simulink model "gm_FFT_DUT"  (R2021a)
settings: Solver=FixedStepDiscrete  StartTime=0.0  StopTime=54  RelTol=1e-3
libraries: simulink x1, dsphdlxfrm x1, dspsrcs4 x1
settings Model: Creator=Tood  LastModifiedBy=Tood
settings SolverCC: AlgebraicLoopSolver=TrustRegion
settings DataIOCC: LimitDataPoints=on  SaveOutput=off  SaveTime=off
settings OptimizationCC: BlockReduction=off  ConditionallyExecuteInputs=off  DefaultParameterBehavior=Inlined  LifeSpan=inf
settings DebuggingCC: AlgebraicLoopMsg=error  InheritedTsInSrcMsg=none  SingleTaskRateTransMsg=error  AllowSymbolicDim=off  StrictBusMsg=ErrorOnBusTreatedAsVector  SFUnexpectedBacktrackingDiag=warning  SFNoUnconditionalDefaultTransitionDiag=warning  SFExecutionAtInitializationDiag=none  SFMachineParentedDataDiag=warning  ArithmeticOperatorsInVariantConditions=warning
settings HardwareCC: ProdBitPerPointer=32  ProdBitPerSizeT=32  ProdBitPerPtrDiffT=32  ProdLargestAtomicFloat=None  ProdIntDivRoundTo=Undefined  ProdEndianess=Unspecified  ProdWordSize=32  ProdHWDeviceType=ASIC/FPGA->ASIC/FPGA  TargetBitPerPointer=64  TargetBitPerSizeT=64  TargetBitPerPtrDiffT=64  TargetLongLongMode=on  TargetIntDivRoundTo=Zero  TargetEndianess=LittleEndian  TargetWordSize=64  TargetHWDeviceType=Custom Processor->MATLAB Host Computer  ProdEqTarget=off
settings SFSimCC: SimUseLocalCustomCode=off  CustomCodeUndefinedFunction=UseInterfaceOnly
settings RTWCC: RTWUseLocalCustomCode=off
settings CodeAppCC: StateflowObjectComments=on
settings GRTTargetCC: TargetLangStandard=C89/C90 (ANSI)
settings ConfigComp: CovScope=ReferencedModels  CovMetricSettings=dw  CovSaveCumulativeToWorkspaceVar=on  CovSaveSingleToWorkspaceVar=on  CovExternalEMLEnable=off  CovSFcnEnable=off

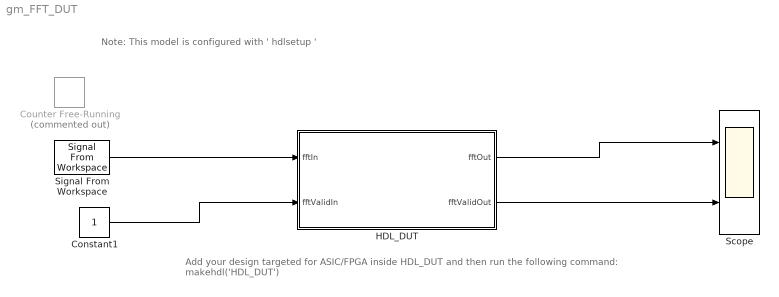
== system gm_FFT_DUT ==
  note: Add your design targeted for ASIC/FPGA inside HDL_DUT and then run the following command:
      | makehdl('HDL_DUT')
  note: Note: This model is configured with ' hdlsetup '
  Constant1 : Constant  OutDataTypeStr=boolean  SampleTime=-1
  Counter Free-Running : simulink/Sources/Counter Free-Running  Commented=on  NumBits=16  tsamp=-1
  HDL_DUT : Subsystem
  Scope : Scope  NumInputPorts=2
  Signal From Workspace : dspsrcs4/Signal From Workspace  X=sig  Ts=1  nsamps=1  OutputAfterFinalValue=Setting to zero  ignoreOrWarnInputAndFrameLengths=off  OutputFrames=off
  wires:
  HDL_DUT/2(fftValidOut) -> Scope/2
  Signal From Workspace/1 -> HDL_DUT/1(fftIn)
  Constant1/1 -> HDL_DUT/2(fftValidIn)
  HDL_DUT/1(fftOut) -> Scope/1

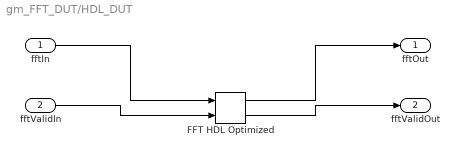
== system gm_FFT_DUT/HDL_DUT ==
  fftIn : Inport  OutDataTypeStr=int16  PortDimensions=1  SampleTime=1
      settings: SignalType=complex
  fftValidIn : Inport  Port=2  OutDataTypeStr=boolean  PortDimensions=1  SampleTime=1
  FFT HDL Optimized : dsphdlxfrm/FFT HDL Optimized  FFTLength=8  Architecture=Streaming Radix 2^2  ComplexMultiplication=Use 3 multipliers and 5 adders  BitReversedOutput=off  BitReversedInput=off  Normalize=off  SimulateUsing=Code generation  RoundingMethod=Round  ResetInputPort=off  StartOutputPort=off  EndOutputPort=off
      settings: SourceProductBaseCode=DS
  fftOut : Outport  SampleTime=1
  fftValidOut : Outport  Port=2  SampleTime=1
  wires:
  fftIn/1 -> FFT HDL Optimized/1
  fftValidIn/1 -> FFT HDL Optimized/2
  FFT HDL Optimized/1 -> fftOut/1
  FFT HDL Optimized/2 -> fftValidOut/1
